simulink model "FCC"  (R2016a)
settings: Solver=VariableStepAuto  StartTime=0.0  StopTime=10.0  RelTol=1e-3
values from neighbouring files (symbols this model uses):
  Xkk = Cin(N*p+N+1:end)    [Controller.m]
  Ymeas = Cin(N*p+1:N*p+N)    [Controller.m]    (also in sample.mat = [2 2 200])
  Yref = reshape(Cin(1:N*p),N,[])    [Controller.m]
settings Model: Creator=hp  LastModifiedBy=hp

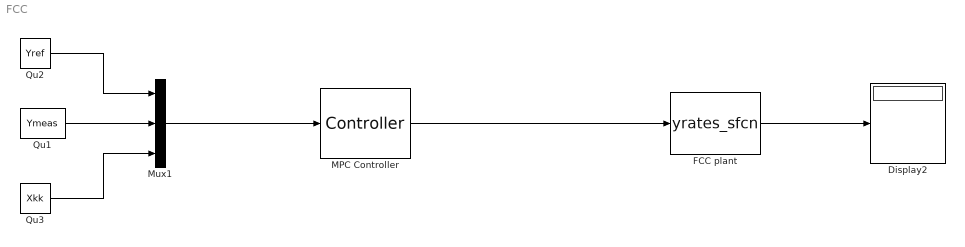
== system FCC ==
  Display2 : Display
  FCC plant : S-Function  FunctionName=yrates_sfcn  Parameters=Y0  SFunctionDeploymentMode=off  EnableBusSupport=off
  MPC Controller : MATLABFcn  MATLABFcn=Controller  Output1D=off
  Mux1 : Mux  Inputs=3
  Qu1 : Constant  Value=Ymeas  VectorParams1D=off
  Qu2 : Constant  Value=Yref  VectorParams1D=off
  Qu3 : Constant  Value=Xkk  VectorParams1D=off
  wires:
  FCC plant/1 -> Display2/1
  Qu2/1 -> Mux1/1
  Qu1/1 -> Mux1/2
  Qu3/1 -> Mux1/3
  Mux1/1 -> MPC Controller/1
  MPC Controller/1 -> FCC plant/1
